simulink model "progetto_simulink"  (R2024b)
settings: Solver=VariableStepAuto  StartTime=0.0  StopTime=T_simulation  RelTol=1e-6
values from neighbouring files (symbols this model uses):
  C = [1 0]    [progetto.m]    (also in progetto_matlab.m)
  DD_test = 0.2    [progetto.m]    (also in progetto_matlab.m)
  NN_test = 0.2    [progetto.m]    (also in progetto_matlab.m)
  omega_d_test = 0.1    [progetto.m]    (also in progetto_matlab.m)
  omega_n_test = 2*10^5    (= 200000)    [progetto.m]    (also in progetto_matlab.m)
  T_star = 0.006    [progetto.m]    (also in progetto_matlab.m)
  u_e = (k*x_1e)/tau(x_1e)    [progetto.m]    (also in progetto_matlab.m)
  WW_test = 2    [progetto.m]    (also in progetto_matlab.m)
  x_1e = deg2rad(140)    [progetto.m]    (also in progetto_matlab.m)
  x_e = [x_1e; x_2e]    [progetto.m]    (also in progetto_matlab.m)
libraries: simulink x2, cstblocks x1
settings Model: Creator=matteolombardi  LastModifiedBy=matteolombardi

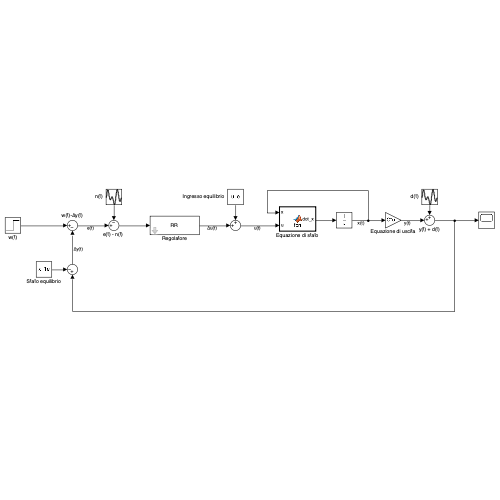
[thumbnail: Simulink's stored preview of the top-level diagram]
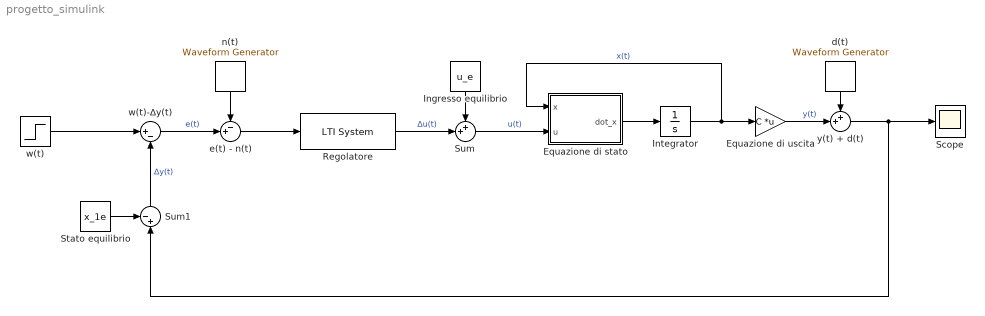
== system progetto_simulink ==
  Equazione di stato : MATLAB Function  TreatAsAtomicUnit=on
  Equazione di uscita : Gain  Gain=C  Multiplication=Matrix(K*u)
  Ingresso equilibrio : Constant  Value=u_e
  Integrator : Integrator  InitialCondition=x_e
  Regolatore : cstblocks/LTI System  sys=RR  IC=[]  PadeOrder=0
  Scope : Scope
  Stato equilibrio : Constant  Value=x_1e
  Sum : Sum  Inputs=++|
  Sum1 : Sum  Inputs=-+|
  d(t) : simulink/Sources/Waveform Generator  OutMin=[]  OutMax=[]  OutDataTypeStr=double  SelectedSignal=1  Signals=sin(DD_test,omega_d_test,0)+sin(DD_test,omega_d_test*2,0)+sin(DD_test,omega_d_test*3,0)+sin(DD_test,omega_d_test*4,0)  BlockNames=MultiportSwitch_9d01a3e6715548a  SampleTime=0.1
  "e(t) - n(t) " : Sum  Inputs=-+|
  n(t) : simulink/Sources/Waveform Generator  OutMin=[]  OutMax=[]  OutDataTypeStr=double  SelectedSignal=1  Signals=sin(NN_test,omega_n_test,0)+sin(NN_test,omega_n_test*2,0)+sin(NN_test,omega_n_test*3,0)+sin(NN_test,omega_n_test*4,0)  BlockNames=MultiportSwitch_8c31f4dd0b14410  SampleTime=0.1
  w(t) : Step  Time=T_star  After=WW_test  SampleTime=0
  w(t)-∆y(t) : Sum  Inputs=|+-
  y(t) + d(t) : Sum  Inputs=++|
  wires:
  Equazione di stato/1(dot_x) -> Integrator/1
  Integrator/1 -> Equazione di uscita/1, Equazione di stato/1(x)  "x(t)"
  Sum/1 -> Equazione di stato/2(u)  "u(t)"
  Ingresso equilibrio/1 -> Sum/1
  Regolatore/1 -> Sum/2  "∆u(t)"
  w(t)/1 -> w(t)-∆y(t)/1
  Sum1/1 -> w(t)-∆y(t)/2  "∆y(t)"
  Stato equilibrio/1 -> Sum1/1
  n(t)/1 -> "e(t) - n(t) "/1
  w(t)-∆y(t)/1 -> "e(t) - n(t) "/2  "e(t)"
  "e(t) - n(t) "/1 -> Regolatore/1
  d(t)/1 -> y(t) + d(t)/1
  Equazione di uscita/1 -> y(t) + d(t)/2  "y(t)"
  y(t) + d(t)/1 -> Sum1/2, Scope/1

== matlab function progetto_simulink/Equazione di stato ==
  data: x input; u input; dot_x output
function dot_x = fcn(x, u)

k     = 1000;
beta  = 0.77;
alpha = deg2rad(25);
J     = 549;

tau = @(theta) cos(alpha)/(1-(sin(alpha)*cos(theta))^2);

dot_x = zeros(2,1);
dot_x(1) = x(2);
dot_x(2) = tau(x(1))/J*u - beta/J*x(2) - k/J*x(1);
